simulink model "HEV_SeriesParallel"  (R2022a)
settings: Solver=ode15s  StartTime=0.0  StopTime=400  RelTol=1e-4  AbsTol=1e-5  EnableMultiTasking=on
PreLoadFcn:
  | load UrbanCycle1
  | load UrbanCycle2
  | load UrbanCycle3
  | load UrbanCycle4
  | load UrbanCycle5
  | 
  | assignin('base','decimation',1)
  | Pbatt = 21e3;
  | Vbatt =100;
  | Ts = 6e-5;   % time step
  | 
  | Drive_Cycle_Num = 1;
  | warning off Simulink:Commands:LoadMdlParameterizedLink
PostLoadFcn:
  | warning off Simulink:Engine:UsingDefaultMaxStepSize
  | warning off Simulink:blocks:MatchingGotoNotFound
  | warning off Simulink:blocks:MatchingFromNotFound
  | warning off Simulink:blocks:TDelayBufferTooSmall
  | warning off Simulink:SL_SaveWithParameterizedLinks_Warning
  | warning off Simulink:SL_TDelayBufferTooSmall
  | warning off Simulink:SL_OutputNotConnected
  | warning off Simulink:SL_SaveWithDisabledLinks_Warning
  | 
  | warning off Simulink:SL_SetParamLinkChangeWarn
  | 
  | warning('off','Simulink:SL_UINotUpdatedDuringRapidAccelSim');
  | warning off Simulink:Engine:OutputNotConnected
  | warning off Simulink:Engine:UINotUpdatedDuringRapidAccelSim
  | warning off Simulink:Engine:SaveWithParameterizedLinks_Warning
  | warning off Simulink:Engine:SolverMaskedZC
  | set_param('HEV_SeriesParallel','MaskedZcDiagnostic','none');
  | warning off Simulink:Engine:SolverInconsistentInitialConditionsWarnForDAE
  | set_param('HEV_SeriesParallel','IgnoredZcDiagnostic','none');
  | warning off Simulink:Engine:SolverIgnoredZCBracketing
  | set_param('HEV_SeriesParallel','MaxConsecutiveZCsMsg','none');
  | warning off Simulink:Engine:SolverConsecutiveZCNum
  | warning off Simulink:Engine:SolverMinStepSizeWarnForDAE
  | warning off Simulink:Engine:SolverMinStepNonlinearIterWarnForDAE
  | warning off simscape:compiler:sli:init:SolverNotRecommended
  | warning off Simulink:Commands:SetParamLinkChangeWarn
  | warning off xPCTarget:sampleTime:sampleTimeInvariance
  | warning off Simulink:blocks:TDelayFixedBuffer
  | 
  | warning('off','physmod:common:gl:sli:rtp:InvalidNonValueReference')
  | warning('off','physmod:common:gl:sli:rtp:InvalidNonValueReferenceMask')
  | 
  | Setup_HEV_Model_Configurations
  | 
  | % Commands to avoid warning at first run
  | % PS battery function
  | warning off MATLAB:illConditionedMatrix
  | try
  |    set_param(bdroot, 'SimulationCommand', 'update');
  | catch
  | end
  | warning on MATLAB:illConditionedMatrix
InitFcn:
  | Configure_HEV_Simulation
StartFcn:
  | tic;
StopFcn:
  | Elapsed_Sim_Time = toc; disp(['Elapsed time for ' bdroot ' = ' num2str(Elapsed_Sim_Time)])
model workspace (MAT data in the model file):
  guiH = 18054.0001221
undefined symbols (not defined in the file or in its folder): Hecate_param1, Hecate_param2, Hecate_param3, Hecate_param4, HEV_Param, sigbuilder_block
libraries: fl_lib x18, nesl_utility x11, HEV_Electrical_Lib x3, sdl_lib x2, HEV_Vehicle_Dynamics_Lib x2, simulink x1, spspowerguiLib x1
(part 2 of 2)

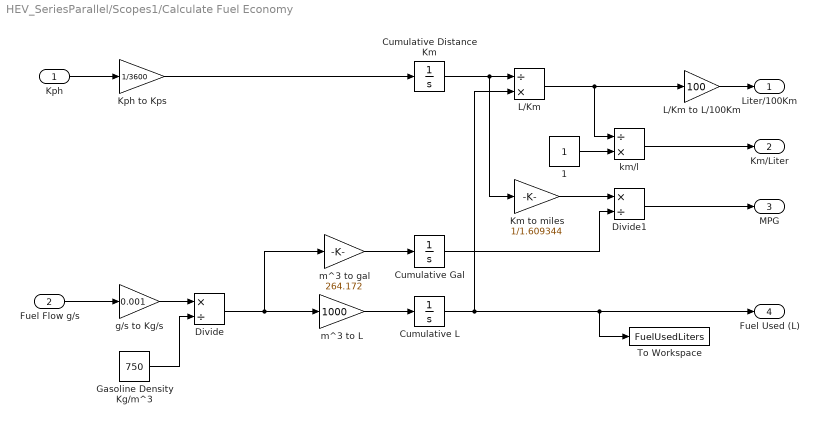
== system HEV_SeriesParallel/Scopes1/Calculate Fuel Economy ==
  Kph : Inport
  Fuel Flow g/s : Inport  Port=2
  1 : Constant
  Cumulative Distance Km : Integrator  InitialCondition=eps
  Cumulative Gal : Integrator  InitialCondition=eps
  Cumulative L : Integrator  InitialCondition=eps
  Divide : Product  Inputs=*/
  Divide1 : Product  Inputs=*/
  Gasoline Density Kg/m^3 : Constant  Value=750
  Km to miles : Gain  Gain=1/1.609344
  Kph to Kps : Gain  Gain=1/3600
  L/Km : Product  Inputs=/*
  L/Km to L/100Km : Gain  Gain=100
  To Workspace : ToWorkspace  VariableName=FuelUsedLiters  SampleTime=-1
      settings: MaxDataPoints=1
  g/s to Kg/s : Gain  Gain=0.001
  km/l : Product  Inputs=/*
  m^3 to L : Gain  Gain=1000
  m^3 to gal : Gain  Gain=264.172
  Liter/100Km : Outport  VectorParamsAs1DForOutWhenUnconnected=off
  Km/Liter : Outport  Port=2  VectorParamsAs1DForOutWhenUnconnected=off
  MPG : Outport  Port=3  VectorParamsAs1DForOutWhenUnconnected=off
  Fuel Used (L) : Outport  Port=4  VectorParamsAs1DForOutWhenUnconnected=off
  wires:
  km/l/1 -> Km/Liter/1
  1/1 -> km/l/2
  Divide1/1 -> MPG/1
  L/Km to L/100Km/1 -> Liter/100Km/1
  Fuel Flow g/s/1 -> g/s to Kg/s/1
  Kph/1 -> Kph to Kps/1
  Cumulative Gal/1 -> Divide1/2
  Km to miles/1 -> Divide1/1
  L/Km/1 -> km/l/1, L/Km to L/100Km/1
  Cumulative Distance Km/1 -> Km to miles/1, L/Km/1
  Cumulative L/1 -> L/Km/2, Fuel Used (L)/1, To Workspace/1
  Kph to Kps/1 -> Cumulative Distance Km/1
  m^3 to gal/1 -> Cumulative Gal/1
  m^3 to L/1 -> Cumulative L/1
  Divide/1 -> m^3 to gal/1, m^3 to L/1
  Gasoline Density Kg/m^3/1 -> Divide/2
  g/s to Kg/s/1 -> Divide/1

== system HEV_SeriesParallel/Speed Sensor/Sensor Dynamics ==
  In : Inport
  Gain : Gain  Gain=1/b
  Integrator : Integrator  InitialCondition=x_initial
  Sum : Sum  Inputs=|+-  InputSameDT=on  SaturateOnIntegerOverflow=on  OutDataTypeStr=Inherit: Same as first input
  Out : Outport  VectorParamsAs1DForOutWhenUnconnected=off
  wires:
  Sum/1 -> Integrator/1
  In/1 -> Sum/1
  Integrator/1 -> Gain/1
  Gain/1 -> Sum/2, Out/1

== system HEV_SeriesParallel/Control/Battery Charge Controller/Inverse engine map ==
  rpm : Inport
  Product : Product  InputSameDT=on  SaturateOnIntegerOverflow=on  OutDataTypeStr=Inherit: Same as first input
  Product1 : Product  Inputs=3  InputSameDT=on  SaturateOnIntegerOverflow=on  OutDataTypeStr=Inherit: Same as first input
  Sum1 : Sum  Inputs=|++  InputSameDT=on  SaturateOnIntegerOverflow=on  OutDataTypeStr=Inherit: Same as first input
  Sum2 : Sum  Inputs=|+-  InputSameDT=on  SaturateOnIntegerOverflow=on  OutDataTypeStr=Inherit: Same as first input
  p1 : Constant  Value=P0/w0
  p2 : Constant  Value=P0/w0^2
  p3 : Constant  Value=P0/w0^3
  rpm2rad/s : Gain  Gain=2*pi/60  SaturateOnIntegerOverflow=on  OutDataTypeStr=Inherit: Same as input  ParamDataTypeStr=Inherit: Same as input
  Tmax : Outport  VectorParamsAs1DForOutWhenUnconnected=off
  wires:
  p1/1 -> Sum1/1
  Sum2/1 -> Tmax/1  "Tmax"
  Product1/1 -> Sum2/2
  Sum1/1 -> Sum2/1
  p3/1 -> Product1/3
  Product/1 -> Sum1/2
  p2/1 -> Product/2
  rpm2rad/s/1 -> Product1/2, Product1/1, Product/1
  rpm/1 -> rpm2rad/s/1

== system HEV_SeriesParallel/Control/Engine Speed Controller/Engine Running ==
  RPM_Dem : Inport
  ICE_Enable : Inport  Port=2
  Alternate Logic : Subsystem
  Select Logic : ManualSwitch
  Engine Running : Outport  VectorParamsAs1DForOutWhenUnconnected=off
  tag scope: engine_running=global
  wires:
  RPM_Dem/1 -> Alternate Logic/1(RPM Dem)
  ICE_Enable/1 -> Select Logic/2
  Alternate Logic/1(ICE Enable) -> Select Logic/1
  Select Logic/1 -> Engine Running/1, [engine_running]

== system HEV_SeriesParallel/Control/Generator Controller/Enable Torque Demand ==
  Gen_Enable : Inport
  TrqDemCtrl : Inport  Port=2
  20Hz Lowpass Filter : TransferFcn  Denominator=[1/(2*pi*20) 1]
  Product : Product  RndMeth=Zero
  Select Logic : ManualSwitch  CurrentSetting=0
  G_Trq_Dem : Outport  VectorParamsAs1DForOutWhenUnconnected=off
  wires:
  Gen_Enable/1 -> 20Hz Lowpass Filter/1
  TrqDemCtrl/1 -> Product/2, Select Logic/2
  20Hz Lowpass Filter/1 -> Product/1
  Select Logic/1 -> G_Trq_Dem/1
  Product/1 -> Select Logic/1

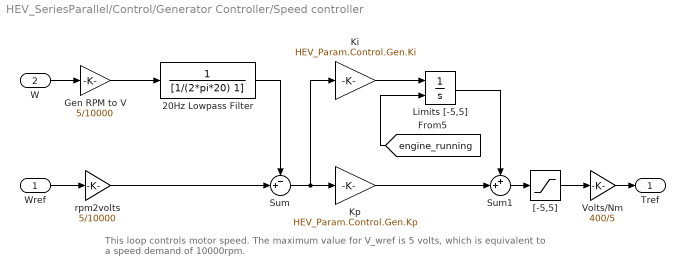
== system HEV_SeriesParallel/Control/Generator Controller/Speed controller ==
  note: This loop controls motor speed. The maximum value for V_wref is 5 volts,
      | which is equivalent to a speed demand of 10000rpm.
  Wref : Inport
  W : Inport  Port=2
  20Hz Lowpass Filter : TransferFcn  Denominator=[1/(2*pi*20) 1]
  Gen RPM to V : Gain  Gain=5/10000
  Ki : Gain  Gain=HEV_Param.Control.Gen.Ki
  Kp : Gain  Gain=HEV_Param.Control.Gen.Kp
  Limits [-5,5] : Integrator  ExternalReset=either  LimitOutput=on  UpperSaturationLimit=5  LowerSaturationLimit=-5
  Sum : Sum  Inputs=-+|
  Sum1 : Sum  Inputs=++|
  Volts/Nm : Gain  Gain=400/5
  "[-5,5]" : Saturate  UpperLimit=5  LowerLimit=-5
  rpm2volts : Gain  Gain=5/10000
  Tref : Outport  VectorParamsAs1DForOutWhenUnconnected=off
  wires:
  Sum/1 -> Ki/1, Kp/1
  [engine_running] -> Limits [-5,5]/2
  20Hz Lowpass Filter/1 -> Sum/1
  Limits [-5,5]/1 -> Sum1/1
  Kp/1 -> Sum1/2
  Ki/1 -> Limits [-5,5]/1
  Sum1/1 -> "[-5,5]"/1
  W/1 -> Gen RPM to V/1
  Wref/1 -> rpm2volts/1
  "[-5,5]"/1 -> Volts/Nm/1
  rpm2volts/1 -> Sum/2
  Gen RPM to V/1 -> 20Hz Lowpass Filter/1
  Volts/Nm/1 -> Tref/1

== system HEV_SeriesParallel/Control/Generator Controller/Subsystem1 ==
  In1 : Inport
  Gen_RPM_Dem : Outport  VectorParamsAs1DForOutWhenUnconnected=off
  tag scope: gen_rpm_dem=global
  wires:
  In1/1 -> Gen_RPM_Dem/1, [gen_rpm_dem]

== system HEV_SeriesParallel/Control/Motor Controller/Enable Torque Demand ==
  Mot_Enable : Inport
  TrqDemCtrl : Inport  Port=2
  20Hz Lowpass Filter : TransferFcn  Denominator=[1/(2*pi*10) 1]
  Product : Product  RndMeth=Zero
  Select Logic : ManualSwitch  CurrentSetting=0
  TrqDem : Outport  VectorParamsAs1DForOutWhenUnconnected=off
  wires:
  Mot_Enable/1 -> 20Hz Lowpass Filter/1
  TrqDemCtrl/1 -> Product/2, Select Logic/2
  Product/1 -> Select Logic/1
  20Hz Lowpass Filter/1 -> Product/1
  Select Logic/1 -> TrqDem/1

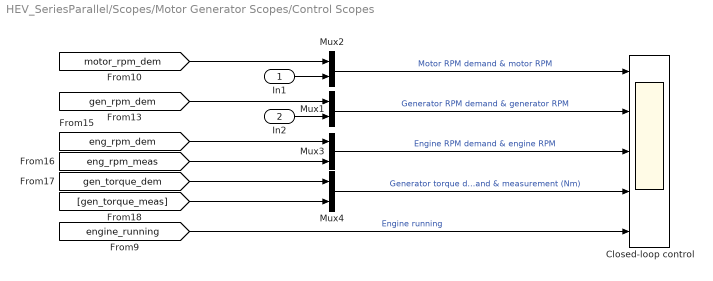
== system HEV_SeriesParallel/Scopes/Motor Generator Scopes/Control Scopes ==
  In1 : Inport
  In2 : Inport  Port=2
  Closed-loop control : Scope  NumInputPorts=5
  Mux{1..4} (4 alike) : Mux  Inputs=2
  wires:
  [motor_rpm_dem] -> Mux2/1
  Mux2/1 -> Closed-loop control/1  "Motor RPM demand & motor RPM"
  [gen_rpm_dem] -> Mux1/1
  Mux1/1 -> Closed-loop control/2  "Generator RPM demand & generator RPM"
  [eng_rpm_dem] -> Mux3/1
  [eng_rpm_meas] -> Mux3/2
  Mux3/1 -> Closed-loop control/3  "Engine RPM demand & engine RPM"
  [gen_torque_dem] -> Mux4/1
  [gen_torque_meas] -> Mux4/2
  Mux4/1 -> Closed-loop control/4  "Generator torque demand & measurement (Nm)"
  [engine_running] -> Closed-loop control/5  "Engine running"
  In1/1 -> Mux2/2
  In2/1 -> Mux1/2

== system HEV_SeriesParallel/Control/Engine Speed Controller/Engine Running/Alternate Logic ==
  RPM Dem : Inport
  Allow time for engine to start : TransportDelay
  No delay for engine stopping : Product  RndMeth=Zero
  Start engine : Fcn  Expr=u(1) > HEV_Param.Control.Engine_Start_RPM
  ICE Enable : Outport  VectorParamsAs1DForOutWhenUnconnected=off
  wires:
  Start engine/1 -> Allow time for engine to start/1, No delay for engine stopping/2
  Allow time for engine to start/1 -> No delay for engine stopping/1
  RPM Dem/1 -> Start engine/1
  No delay for engine stopping/1 -> ICE Enable/1

== stateflow chart HEV_SeriesParallel/FitnessConverter_Hecate ==
  state step_1
    fitness_1 = Inf;
    fitness_2 = Inf;
  state step_2
    fitness_1 = 1.5-(speed_o_delta);
    fitness_2 = Inf;
  state step_3
    fitness_1 = Inf;
    fitness_2 = 1-(speed_o_delta);
  (default) -> step_1
  step_3 -> step_1 : [after(90,sec)]
  step_1 -> step_2 : [after(1,sec)]
  step_2 -> step_3 : [after(9,sec)]
  data: speed_o_delta input; fitness_1 output; fitness_2 output

== stateflow chart HEV_SeriesParallel/Test Sequence ==
  state step_1
    Speed_Demand=Hecate_param1;
    %Speed_Demand=4;
  state step_2
    Speed_Demand=Hecate_param2;
    %Speed_Demand=0;
  state step_3
    Speed_Demand=Hecate_param3;
    %Speed_Demand=4;
  state step_4
    Speed_Demand=Hecate_param4;
    %Speed_Demand=0;
  (default) -> step_1
  step_1 -> step_2 : [
      | after(100,sec)
      | ]
  step_2 -> step_3 : [
      | after(100,sec)
      | ]
  step_3 -> step_4 : [
      | after(100,sec)
      | ]
  data: Speed_Demand output; Hecate_param1 parameter; Hecate_param2 parameter; Hecate_param3 parameter; Hecate_param4 parameter

== stateflow chart HEV_SeriesParallel/Test Assessment ==
  state step_1
  state step_2
    verify(speed_o_delta<1.5)
  state step_3
    verify(speed_o_delta<1)
  (default) -> step_1
  (junction 63) -> step_1
  (junction 65) -> (junction 63)
  step_1 -> step_2 : [
      | after(1,sec)
      | ]
  step_2 -> step_3 : [
      | after(9,sec)
      | ]
  step_3 -> (junction 65) : [
      | after(90,sec)
      | ]
  data: speed_o_delta input

== stateflow chart HEV_SeriesParallel/Control/Mode Logic ==
  settings: updateMethod=DISCRETE  sampleTime=HEV_Param.Control.Mode_Logic_TS
  state Motion_mode
    state Start_mode
      entry: Gen_Enable=1;
      Mot_Enable=1;
      ICE_Enable=0;
    state Normal_mode
      entry: ICE_Enable=1;
      state Accelerate_mode
        entry: Gen_Enable=0;
        Mot_Enable=1;
      state Cruise_mode
        entry: Mot_Enable=1;
        state charge
          entry:Gen_Enable=1;
        state nocharge
          entry:Gen_Enable=0;
        (default) -> charge
        charge -> nocharge : [charge>99.9]
        nocharge -> charge : [charge<30]
      (default) -> Accelerate_mode
      Cruise_mode -> Accelerate_mode : [(speed <0.998*oldspeed() ...
          | || speed>1.002*oldspeed()) ...
          | && charge>30]
      Accelerate_mode -> Cruise_mode : [(speed >0.998*oldspeed() ...
          |  && speed<1.002* ...
          | oldspeed())|| charge<=30]
    (default) -> Start_mode
    Normal_mode -> Start_mode : [engine_speed<=EngOffRPM]
    Start_mode -> Normal_mode : [engine_speed>EngOnRPM]
  state Brake_mode
    entry: Mot_Enable=1;
    Gen_Enable=0;
    ICE_Enable=0;
  (default) -> Motion_mode
  Motion_mode -> Brake_mode : [brake>=0.05]
  Brake_mode -> Motion_mode : [brake<0.05]
  data: y function_output double; speed input; Mot_Enable output double; Gen_Enable output double; brake input; speed_buffer local double size=21; ICE_Enable output double; charge input; engine_speed input; EngOnRPM constant double =HEV_Param.Control.Engine_Start_RPM; EngOffRPM constant double =HEV_Param.Control.Engine_Stop_RPM
  function y = oldspeed:
    | function y = oldspeed
    | speed_buffer(2:end) = speed_buffer(1:end-1);
    | speed_buffer(1) = speed;
    | y = mean(speed_buffer);
